simulink model "Fan"  (R2023a)
settings: Solver=VariableStepAuto  StartTime=0.0  StopTime=10.0  RelTol=1e-3  AbsTol=1e-3
model workspace (MAT data in the model file):
  Fan.shaftspeed = [14400 15600 16800 18000 19200 20400 21600 22800 24000 25200 26400 27600 28800 30000 31200 32400 33600 34800 36000 37200 38400 39600 40800 42000 43200 44400 45600 46800 48000]
  Fan.presstable = [0; 1; 2; 3; 4; 5; 6; 7; 8]
  Fan.flowvector = [97.5714285714 106 114 122 128.666666667 137 147.5 160.272727273 169.5 178.424242424 186.909090909 195.25 ... (261 elements, 29x9)]
  Fan.efficiency = [0.45  0.45  NaN  NaN  NaN  NaN  NaN  NaN  NaN; 0.45  0.45  NaN  NaN  NaN  NaN  NaN  NaN  NaN; 0.45  0.45  NaN  NaN  NaN  NaN  NaN  NaN  NaN; 0.45  0.45  NaN  NaN  NaN  NaN  NaN  NaN  NaN; 0.45  0.45  NaN  NaN  NaN  NaN  NaN  NaN  NaN; 0.45  0.45  NaN  NaN  NaN  NaN  NaN  NaN  NaN; 0.45  0.45  0.45  NaN  NaN  NaN  NaN  NaN  NaN; 0.45  0.45  0.45  NaN  NaN  NaN  NaN  NaN  NaN; 0.45  0.45  0.45  0.45  NaN  NaN  NaN  NaN  NaN; 0.45  0.45  0.45  0.45  NaN  NaN  NaN  NaN  NaN; 0.45  0.45  0.45  0.45  NaN  NaN  NaN  NaN  NaN; 0.45  0.45  0.45  0.45  NaN  NaN  NaN  NaN  NaN; 0.45  0.45  0.45  0.45  NaN  NaN  NaN  NaN  NaN; 0.45  0.45  0.45  0.45  0.45  NaN  NaN  NaN  NaN; 0.45  0.45  0.45  0.45  0.45  NaN  NaN  NaN  NaN; 0.45  0.45  0.45  0.45  0.45  NaN  NaN  NaN  NaN; 0.45  0.45  0.45  0.45  0.45  0.45  NaN  NaN  NaN; 0.45  0.45  0.45  0.45  0.45  0.45  NaN  NaN  NaN; 0.45  0.45  0.45  0.45  0.45  0.45  0.45  NaN  NaN; 0.45  0.45  0.45  0.45  0.45  0.45  0.45  NaN  NaN; 0.45  0.45  0.45  0.45  0.45  0.45  0.45  NaN  NaN; 0.45  0.45  0.45  0.45  0.45  0.45  0.45  NaN  NaN; 0.45  0.45  0.45  0.45  0.45  0.45  0.45  0.45  NaN; 0.45  0.45  0.45  0.45  0.45  0.45  0.45  0.45  NaN; 0.45  0.45  0.45  0.45  0.45  0.45  0.45  0.45  NaN; 0.45  0.45  0.45  0.45  0.45  0.45  0.45  0.45  0.45; 0.45  0.45  0.45  0.45  0.45  0.45  0.45  0.45  0.45; 0.45  0.45  0.45  0.45  0.45  0.45  0.45  0.45  0.45; 0.45  0.45  0.45  0.45  0.45  0.45  0.45  0.45  0.45]
  Pipe.area = 0.000314159265359
  Pipe.longlength = 0.1
  Pipe.shortlength = 0.05
libraries: fl_lib x10, nesl_utility x4, SimscapeFluids_lib x1
(part 1 of 3)
settings Model: Creator=xuluyu  LastModifiedBy=xuluyu
settings SolverCC: AutoScaleAbsTol=off  AlgebraicLoopSolver=TrustRegion  MaxZcPerStep=1
settings DebuggingCC: UnconnectedInputMsg=warning  UnconnectedOutputMsg=warning  UnconnectedLineMsg=warning  SymbolicDimsDataTypeCodeGenerationDiagnostic=none
settings ModelReferenceCC: EnableRefExpFcnMdlSchedulingChecks=on
settings SFSimCC: CustomCodeUndefinedFunction=UseInterfaceOnly
settings RTWCC: DLArmComputeVersion=19.05
settings SimscapeCC: SimscapeLogType=all  SimscapeLogSimulationStatistics=on  SimscapeLogOpenViewer=on  SimscapeLogDataHistory=10000

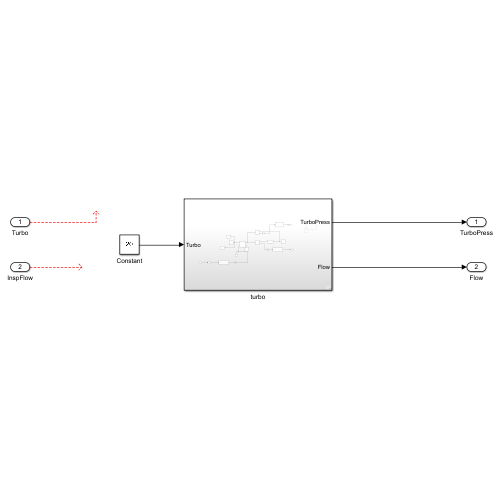
[thumbnail: Simulink's stored preview of the top-level diagram]
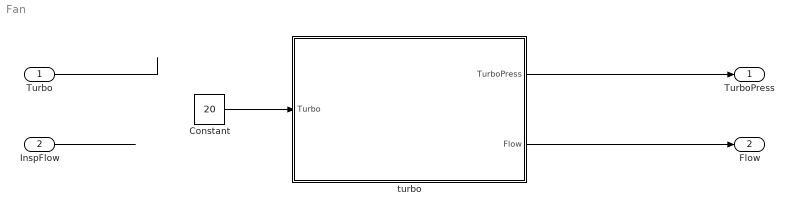
== system Fan ==
  Turbo : Inport
  InspFlow : Inport  Port=2
  Constant : Constant  Value=20
  turbo : Subsystem
  TurboPress : Outport
  Flow : Outport  Port=2
  wires:
  Turbo/1 -> ?
  InspFlow/1 -> ?
  turbo/1(TurboPress) -> TurboPress/1
  Constant/1 -> turbo/1(Turbo)
  turbo/2(Flow) -> Flow/1
